simulink model "State_space_feedback"  (R2023a)
settings: Solver=VariableStepAuto  StartTime=0.0  StopTime=20  RelTol=1e-3
values from neighbouring files (symbols this model uses):
  A = [0                 1   0                                              0 ... (first row only)    [State_space_feedback.m]    (also in state feedback and PID and root locus.m)
  B = L/N    (= 0.111111111111)    [State_space_feedback.m]    (also in generate_road_profile.m; state feedback and PID and root locus.m = [0                 0)
settings Model: Creator=Abdulrahman Hamdy  LastModifiedBy=Abderrahman

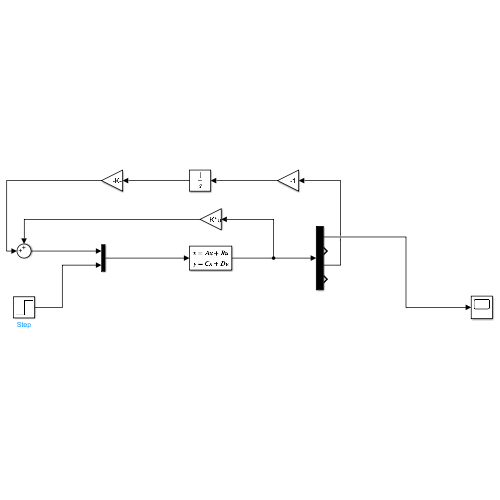
[thumbnail: Simulink's stored preview of the top-level diagram]
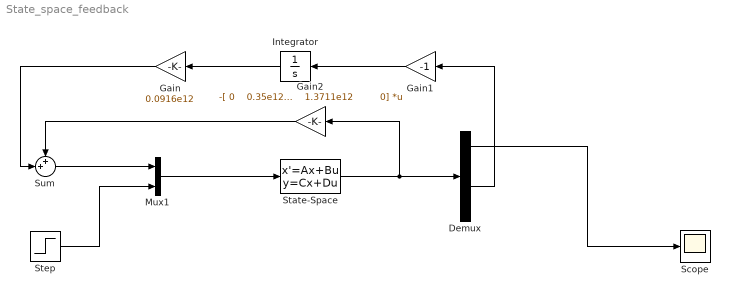
== system State_space_feedback ==
  Demux : Demux
  Gain : Gain  Gain=0.0916e12
  Gain1 : Gain  Gain=-1
  Gain2 : Gain  Gain="-[ 0    0.35e12    1.3711e12         0]"  Multiplication=Matrix(K*u)
  Integrator : Integrator
  Mux1 : Mux  Inputs=2
  Scope : Scope
  State-Space : StateSpace  A=A  B=B  C=eye(4)  D=zeros(4,2)  InitialCondition=0  ParameterTunability=Unconstrained
  Step : Step  SampleTime=0
  Sum : Sum  Inputs=++|
  wires:
  Mux1/1 -> State-Space/1
  Step/1 -> Mux1/2
  Integrator/1 -> Gain/1
  Gain1/1 -> Integrator/1
  Sum/1 -> Mux1/1
  Gain2/1 -> Sum/1
  State-Space/1 -> Gain2/1, Demux/1
  Gain/1 -> Sum/2
  Demux/3 -> Gain1/1
  Demux/1 -> Scope/1
